simulink model "Saturation"  (R2020b)
settings: Solver=VariableStepAuto  StartTime=0.0  StopTime=80  RelTol=1e-3
settings Model: Creator=luke  LastModifiedBy=luke

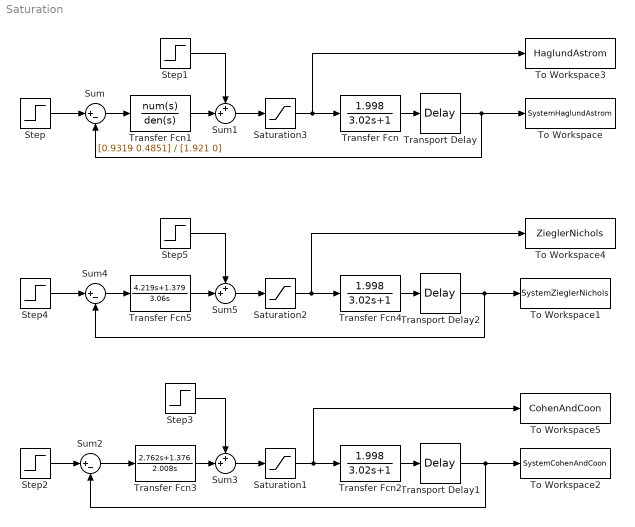
== system Saturation ==
  Saturation1 : Saturate  UpperLimit=0.75  LowerLimit=-0.75
  Saturation2 : Saturate  UpperLimit=0.75  LowerLimit=-0.75
  Saturation3 : Saturate  UpperLimit=0.75  LowerLimit=-0.75
  Step : Step  SampleTime=0
  Step1 : Step  Time=40  SampleTime=0
  Step2 : Step  SampleTime=0
  Step3 : Step  Time=40  SampleTime=0
  Step4 : Step  SampleTime=0
  Step5 : Step  Time=40  SampleTime=0
  Sum : Sum  Inputs=|+-
  Sum1 : Sum  Inputs=++|
  Sum2 : Sum  Inputs=|+-
  Sum3 : Sum  Inputs=++|
  Sum4 : Sum  Inputs=|+-
  Sum5 : Sum  Inputs=++|
  To Workspace : ToWorkspace  VariableName=SystemHaglundAstrom  SaveFormat=Timeseries  SampleTime=0.0001
  To Workspace1 : ToWorkspace  VariableName=SystemZieglerNichols  SaveFormat=Timeseries  SampleTime=0.0001
  To Workspace2 : ToWorkspace  VariableName=SystemCohenAndCoon  SaveFormat=Timeseries  SampleTime=0.0001
  To Workspace3 : ToWorkspace  VariableName=HaglundAstrom  SaveFormat=Timeseries  SampleTime=0.0001
  To Workspace4 : ToWorkspace  VariableName=ZieglerNichols  SaveFormat=Timeseries  SampleTime=0.0001
  To Workspace5 : ToWorkspace  VariableName=CohenAndCoon  SaveFormat=Timeseries  SampleTime=0.0001
  Transfer Fcn : TransferFcn  Numerator=[1.998]  Denominator=[3.02 1]
  Transfer Fcn1 : TransferFcn  Numerator=[0.9319 0.4851]  Denominator=[1.921 0]
  Transfer Fcn2 : TransferFcn  Numerator=[1.998]  Denominator=[3.02 1]
  Transfer Fcn3 : TransferFcn  Numerator=[2.762 1.376]  Denominator=[2.008 0]
  Transfer Fcn4 : TransferFcn  Numerator=[1.998]  Denominator=[3.02 1]
  Transfer Fcn5 : TransferFcn  Numerator=[4.219 1.379]  Denominator=[3.06 0]
  Transport Delay : TransportDelay  BufferSize=10240
  Transport Delay1 : TransportDelay  BufferSize=10240
  Transport Delay2 : TransportDelay  BufferSize=10240
  wires:
  Step/1 -> Sum/1
  Sum/1 -> Transfer Fcn1/1
  Step1/1 -> Sum1/1
  Sum2/1 -> Transfer Fcn3/1
  Step2/1 -> Sum2/1
  Step3/1 -> Sum3/1
  Sum4/1 -> Transfer Fcn5/1
  Step4/1 -> Sum4/1
  Step5/1 -> Sum5/1
  Saturation3/1 -> Transfer Fcn/1, To Workspace3/1
  Sum1/1 -> Saturation3/1
  Transfer Fcn/1 -> Transport Delay/1
  Sum5/1 -> Saturation2/1
  Saturation2/1 -> Transfer Fcn4/1, To Workspace4/1
  Transfer Fcn4/1 -> Transport Delay2/1
  Sum3/1 -> Saturation1/1
  Saturation1/1 -> Transfer Fcn2/1, To Workspace5/1
  Transfer Fcn2/1 -> Transport Delay1/1
  Transfer Fcn5/1 -> Sum5/2
  Transfer Fcn1/1 -> Sum1/2
  Transfer Fcn3/1 -> Sum3/2
  Transport Delay/1 -> Sum/2, To Workspace/1
  Transport Delay2/1 -> To Workspace1/1, Sum4/2
  Transport Delay1/1 -> Sum2/2, To Workspace2/1
